simulink model "balanceActual"  (R2012b)
settings: Solver=ode3  StartTime=0.0  StopTime=inf  FixedStep=0.001  RelTol=1e-3
undefined symbols (not defined in the file or in its folder): HIL, qc_get_step_size
libraries: quarc_library x7
settings Model: SimulationMode=external  ExtModeTrigDuration=15000  Creator=runkunwang  LastModifiedBy=runkunwang
settings SolverCC: PositivePriorityOrder=on
settings RTWCC: SystemTargetFile=quarc_win64.tlc  TemplateMakefile=quarc_default_tmf  Description=QUARC Win64 Target  ProcessScript=quarc_win64_make_rtw_hook
settings STFCustomTargetCC: TargetPreCompLibLocation=C:\PROGRA~3\QUARC\lib\2012b\win64\release  CodeReplacementLibrary=ANSI_C  GeneratePreprocessorConditionals=Disable all  CombineOutputUpdateFcns=on  GRTInterface=off  SystemTargetFile=quarc_win64.tlc
settings GRTTargetCC: TargetPreCompLibLocation=C:\PROGRA~3\QUARC\lib\2012b\win64\release  ParMdlRefBuildCompliant=off  CompOptLevelCompliant=off  ConcurrentExecutionCompliant=off  MatFileLogging=off  ExtMode=on  ExtModeMexFile=quarc_comm

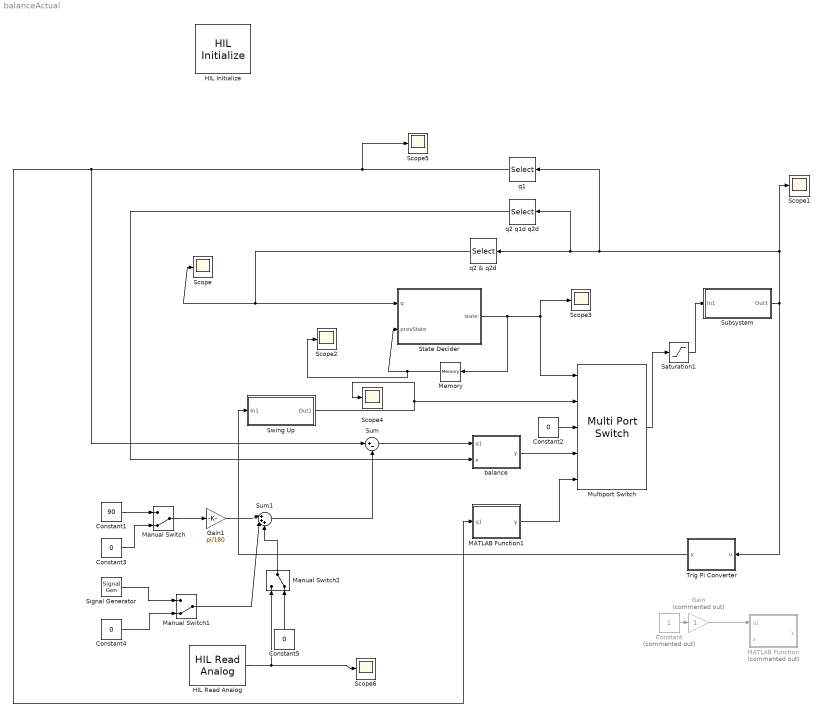
== system balanceActual ==
  Constant : Constant  Commented=on
  Constant1 : Constant  Value=90
  Constant{2..5} (4 alike) : Constant  Value=0
  Gain : Gain  Commented=on
  Gain1 : Gain  Gain=pi/180
  HIL Initialize : quarc_library/Data Acquisition/Generic/Configuration/HIL Initialize  Priority=-99  object_name=HIL-1  board_type=q2_usb  board_number=0  board_options=d0=digital;d1=digital;led=auto;update_rate=normal;decimation=1  exclusive=off  active=off  hardware_clocks=[0]  clock_modes=[]  initial_clock_frequencies=[]  set_clock_params_at_start=off  set_clock_params_at_switch_in=off  set_clock_frequencies_at_start=off  set_clock_frequencies_at_switch_in=off  analog_input_channels=[0:1]  analog_input_maximums=10  analog_input_minimums=-10  set_analog_input_params_at_start=on  set_analog_input_params_at_switch_in=off  analog_output_channels=[0:1]  analog_output_maximums=10  analog_output_minimums=-10  initial_analog_outputs=[0]  final_analog_outputs=[0]  watchdog_analog_outputs=0  set_analog_output_params_at_start=on  set_analog_output_params_at_switch_in=off  set_analog_outputs_at_start=on  set_analog_outputs_at_switch_in=off  set_analog_outputs_at_terminate=on  set_analog_outputs_at_switch_out=off  set_analog_outputs_on_watchdog=off  digital_input_channels=[]  digital_output_channels=[]  digital_output_configuration=[]  initial_digital_outputs=[1]  final_digital_outputs=[1]  watchdog_digital_outputs=[1]  set_digital_output_params_at_start=off  set_digital_output_params_at_switch_in=off  set_digital_outputs_at_start=on  set_digital_outputs_at_switch_in=off  set_digital_outputs_at_terminate=on  set_digital_outputs_at_switch_out=off  set_digital_outputs_on_watchdog=off  encoder_channels=[0:1]  quadrature=[4]  encoder_filter_frequency=[]  initial_encoder_counts=[0]  set_encoder_params_at_start=on  set_encoder_params_at_switch_in=off  set_encoder_counts_at_start=on  set_encoder_counts_at_switch_in=off  pwm_channels=[]  pwm_modes=[0]  pwm_frequency=1/0.020  pwm_configuration=[]  pwm_alignment=[]  pwm_polarity=[]  pwm_leading_deadband=[]  pwm_trailing_deadband=[]  initial_pwm_outputs=[0]  final_pwm_outputs=[0]  watchdog_pwm_outputs=[0]  set_pwm_params_at_start=on  set_pwm_params_at_switch_in=off  set_pwm_outputs_at_start=on  set_pwm_outputs_at_switch_in=off  set_pwm_outputs_at_terminate=on  set_pwm_outputs_at_switch_out=off  set_pwm_outputs_on_watchdog=off  other_output_channels=[]  initial_other_outputs=[]  final_other_outputs=[]  watchdog_other_outputs=[]  set_other_outputs_at_start=off  set_other_outputs_at_switch_in=off  set_other_outputs_at_terminate=off  set_other_outputs_at_switch_out=off  set_other_outputs_on_watchdog=off
  HIL Read Analog : quarc_library/Data Acquisition/Generic/Immediate I//O/HIL Read Analog  object_name=HIL-1  channels=0  sample_time=qc_get_step_size  active=on  vector_output=off
  MATLAB Function : MATLAB Function  Commented=on  TreatAsAtomicUnit=on
  MATLAB Function1 : MATLAB Function  TreatAsAtomicUnit=on
  Manual Switch : ManualSwitch  CurrentSetting=0
  Manual Switch1 : ManualSwitch  CurrentSetting=0
  Manual Switch2 : ManualSwitch  CurrentSetting=0
  Memory : Memory  X0=1
  Multiport Switch : MultiPortSwitch  Inputs=4
  Saturation1 : Saturate  UpperLimit=10  LowerLimit=-10
  Scope{,1..6} (7 alike) : Scope
      Scope settings: YMin=-0.5  YMax=9.5
      Scope1 settings: YMin=-0.6  YMax=0.7
      Scope2 settings: SaveName=ScopeData2  MaxDataPoints=10000
      Scope3 settings: SaveName=ScopeData3  MaxDataPoints=10000
      Scope4 settings: SaveName=ScopeData4  MaxDataPoints=10000
      Scope5 settings: YMin=-0.5  YMax=9.5  SaveName=ScopeData5
      Scope6 settings: SaveName=ScopeData6
  Signal Generator : SignalGenerator  Amplitude=50  Frequency=0.1
  State Decider : MATLAB Function  TreatAsAtomicUnit=on
  Subsystem : Subsystem
  Sum : Sum  Inputs=|+-
  Sum1 : Sum  Inputs=|+++
  Swing Up : Subsystem
  Trig Pi Converter : MATLAB Function  TreatAsAtomicUnit=on
  balance : MATLAB Function  TreatAsAtomicUnit=on
  q1 : Selector  InputPortWidth=4  IndexOptions=Index vector (dialog)  Indices=[1]  OutputSizes=1
  q2 & q2d : Selector  InputPortWidth=4  IndexOptions=Index vector (dialog)  Indices=[1 3 4]  OutputSizes=1
  q2 q1d q2d : Selector  InputPortWidth=4  IndexOptions=Index vector (dialog)  Indices=[2 3 4]  OutputSizes=1
  wires:
  State Decider/1(state) -> Memory/1, Multiport Switch/1, Scope3/1
  Constant2/1 -> Multiport Switch/3
  q2 & q2d/1 -> Scope/1, State Decider/1(q)
  Multiport Switch/1 -> Saturation1/1
  Saturation1/1 -> Subsystem/1(In1)
  Memory/1 -> Scope2/1, State Decider/2(prevState)
  Swing Up/1(Out1) -> Scope4/1, Multiport Switch/2
  Subsystem/1(Out1) -> Trig Pi Converter/1(u), Scope1/1, q1/1, q2 q1d q2d/1, q2 & q2d/1
  Trig Pi Converter/1(y) -> Swing Up/1(In1)
  balance/1(y) -> Multiport Switch/4
  Constant/1 -> Gain/1
  Gain/1 -> MATLAB Function/1(q1)
  q2 q1d q2d/1 -> balance/2(x)
  q1/1 -> MATLAB Function1/1(q1), Sum/1, Scope5/1
  Sum/1 -> balance/1(q1)
  Constant1/1 -> Manual Switch/1
  Constant3/1 -> Manual Switch/2
  Signal Generator/1 -> Manual Switch1/1
  Constant4/1 -> Manual Switch1/2
  Manual Switch1/1 -> Sum1/2
  MATLAB Function1/1(y) -> Multiport Switch/5
  Manual Switch/1 -> Gain1/1
  Gain1/1 -> Sum1/1
  Sum1/1 -> Sum/2
  HIL Read Analog/1 -> Manual Switch2/1, Scope6/1
  Manual Switch2/1 -> Sum1/3
  Constant5/1 -> Manual Switch2/2

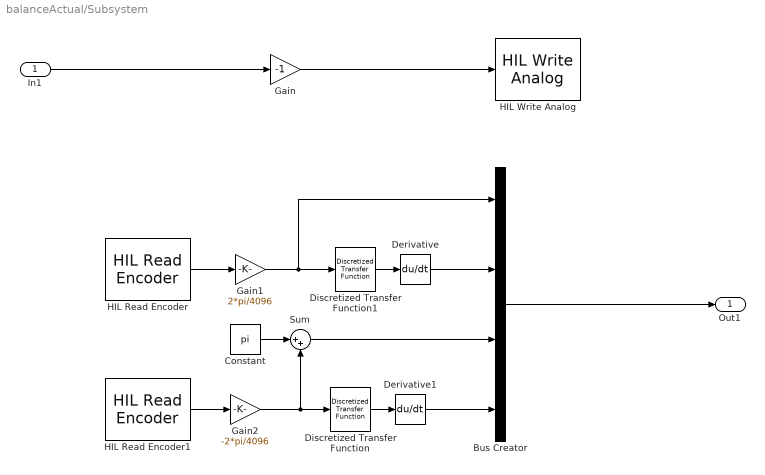
== system balanceActual/Subsystem ==
  In1 : Inport
  Bus Creator : BusCreator
  Constant : Constant  Value=pi
  Derivative : Derivative
  Derivative1 : Derivative
  Discretized Transfer Function : quarc_library/Discrete/Discretized Transfer Function  num=100  den=[1 100]  method=tustin  Ts=qc_get_step_size
  Discretized Transfer Function1 : quarc_library/Discrete/Discretized Transfer Function  num=100  den=[1 100]  method=tustin  Ts=qc_get_step_size
  Gain : Gain  Gain=-1
  Gain1 : Gain  Gain=2*pi/4096  ParamMin=[-512]  ParamMax=[512]
  Gain2 : Gain  Gain=-2*pi/4096  ParamMin=[-512]  ParamMax=[512]
  HIL Read Encoder : quarc_library/Data Acquisition/Generic/Immediate I//O/HIL Read Encoder  object_name=HIL-1  channels=0  sample_time=qc_get_step_size  active=on  vector_output=off  data_type_mode=Inherit via back propagation  data_type=double
  HIL Read Encoder1 : quarc_library/Data Acquisition/Generic/Immediate I//O/HIL Read Encoder  object_name=HIL-1  channels=1  sample_time=qc_get_step_size  active=on  vector_output=off  data_type_mode=Inherit via back propagation  data_type=double
  HIL Write Analog : quarc_library/Data Acquisition/Generic/Immediate I//O/HIL Write Analog  object_name=HIL-1  channels=0  sample_time=-1  active=off  vector_input=off
  Sum : Sum  Inputs=|++
  Out1 : Outport
  wires:
  HIL Read Encoder/1 -> Gain1/1
  HIL Read Encoder1/1 -> Gain2/1
  Gain1/1 -> Bus Creator/1, Discretized Transfer Function1/1
  Gain2/1 -> Discretized Transfer Function/1, Sum/2
  Discretized Transfer Function1/1 -> Derivative/1
  Discretized Transfer Function/1 -> Derivative1/1
  Constant/1 -> Sum/1
  In1/1 -> Gain/1
  Gain/1 -> HIL Write Analog/1
  Bus Creator/1 -> Out1/1
  Derivative/1 -> Bus Creator/2
  Sum/1 -> Bus Creator/3
  Derivative1/1 -> Bus Creator/4

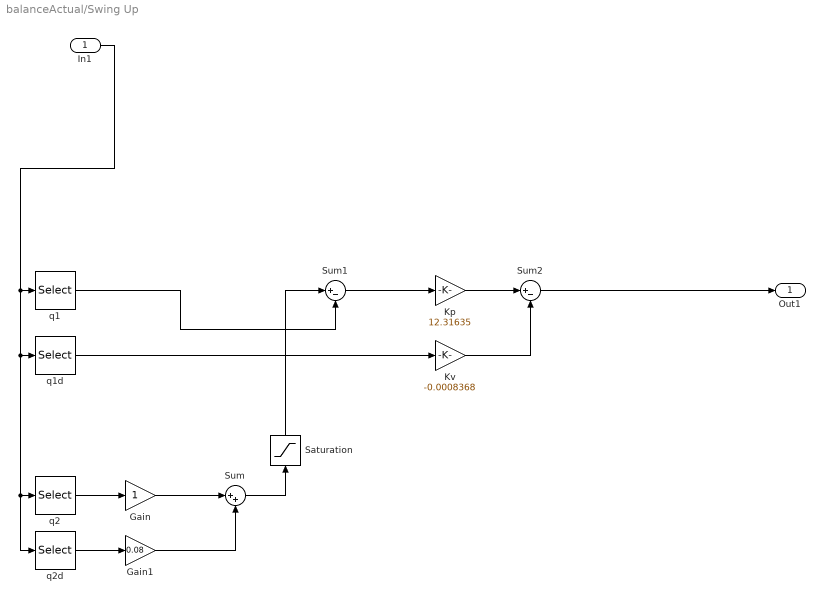
== system balanceActual/Swing Up ==
  In1 : Inport
  Gain : Gain
  Gain1 : Gain  Gain=0.08
  Kp : Gain  Gain=12.31635
  Kv : Gain  Gain=-0.0008368
  Saturation : Saturate
  Sum : Sum  Inputs=|++
  Sum1 : Sum  Inputs=|+-
  Sum2 : Sum  Inputs=|+-
  q1 : Selector  InputPortWidth=4  IndexOptions=Index vector (dialog)  Indices=[1]  OutputSizes=1
  q1d : Selector  InputPortWidth=4  IndexOptions=Index vector (dialog)  Indices=[2]  OutputSizes=1
  q2 : Selector  InputPortWidth=4  IndexOptions=Index vector (dialog)  Indices=[3]  OutputSizes=1
  q2d : Selector  InputPortWidth=4  IndexOptions=Index vector (dialog)  Indices=[4]  OutputSizes=1
  Out1 : Outport
  wires:
  In1/1 -> q2d/1, q2/1, q1d/1, q1/1
  q1d/1 -> Kv/1
  q2/1 -> Gain/1
  q2d/1 -> Gain1/1
  Gain/1 -> Sum/1
  Gain1/1 -> Sum/2
  Sum1/1 -> Kp/1
  Kv/1 -> Sum2/2
  Kp/1 -> Sum2/1
  Sum2/1 -> Out1/1
  Sum/1 -> Saturation/1
  q1/1 -> Sum1/2
  Saturation/1 -> Sum1/1

== matlab function balanceActual/Trig Pi Converter ==
  data: u input; y output
function y = fcn(u)
q1 = u(1);
q1d = u(2);
q2d = u(4);
q2 = u(3);
q2 = q2 - pi;
y = [q1 q1d atan2(sin(q2),cos(q2)) q2d];

== matlab function balanceActual/State Decider ==
  data: q input; state output; prevState input
function state = fcn(q, prevState)
q1 = q(1);
q2 = q(2);
q2d = q(3);
q2 = q2 - pi;

%q1 mod
if q1 < 0
    q1 = -q1;
end
if q1 > 2*pi
    q1 = mod(q1, 2*pi);
end

%q2 mod
if q2 < 0
    q2 = -q2;
end
if q2 > 2*pi
    q2 = mod(q2, 2*pi);
end

%controller starts
%Zone 1 to Zone 3
if prevState == 1 && (q2 > (8*pi)/9 && q2 < (10*pi)/9)
    %Zone 3
    state = 3;
%Zone 3 to Zone 2
elseif prevState == 3 && (q2 < (8*pi)/9 || q2 > (10*pi)/9)
    %Zone 2
    state = 2; 
%Fourth State to Zone 1
elseif prevState == 4 && (q2 < (pi/18) && q2 < (35*pi/18)) && (abs(q2d) < 1) && (q1 < pi/18 || q1 > 35*pi/18)
    %Zone 1
    state = 1; 

%fourth state
elseif prevState == 2 && (q2 < (pi/18) && q2 < (35*pi/18)) && (abs(q2d) < 1) && q1 ~= 0
    %State 4
    state = 4;
%Zone 2 to Zone 1
    
else state = prevState;
end

end

== matlab function balanceActual/MATLAB Function ==
  data: q1 input; y output; x input
function y = fcn(q1, x)

%theta values
t1 = 0.0790;
t2 = 0.0277;
t3 = 0.0278;
t4 = 0.1347;
t5 = 0.5397;
t6 = 0.0057;

%actual position
q1a = x(1);
q2a = x(3);
q1da = x(2);
q2da = x(4);
q2n = atan2(sin(q2a),cos(q2a));

%desired positions
q2 = 0;
q1d = 0;
q2d = 0;
%A matrx
A = zeros(4);
A(1,2) = 1;
A(3,4) = 1;
A(2,2) = - (t2*(t5 + 2*q2d*t2*cos(q2)*sin(q2)))/(t1*t2 - t3^2*cos(q2)^2 + t2^2*sin(q2)^2) - (2*q1d*t2*t3*cos(q2)^2*sin(q2))/(t1*t2 - t3^2*cos(q2)^2 + t2^2*sin(q2)^2);
A(2,3) = (t2*(q2d^2*t3*cos(q2) - 2*q1d*q2d*t2*cos(q2)^2 + 2*q1d*q2d*t2*sin(q2)^2))/(t1*t2 - t3^2*cos(q2)^2 + t2^2*sin(q2)^2) - (t3*cos(q2)*((981*t4*cos(q2))/100 + q1d^2*t2*cos(q2)^2 - q1d^2*t2*sin(q2)^2))/(t1*t2 - t3^2*cos(q2)^2 + t2^2*sin(q2)^2) + (t3*sin(q2)*(t2*cos(q2)*sin(q2)*q1d^2 - q2d*t6 + (981*t4*sin(q2))/100))/(t1*t2 - t3^2*cos(q2)^2 + t2^2*sin(q2)^2) - (t2*(2*cos(q2)*sin(q2)*t2^2 + 2*cos(q2)*sin(q2)*t3^2)*(t3*sin(q2)*q2d^2 - 2*q1d*t2*cos(q2)*sin(q2)*q2d + v - q1d*t5))/(t2^2*sin(q2)^2 + t1*t2 - t3^2*cos(q2)^2)^2 + (t3*cos(q2)*(2*cos(q2)*sin(q2)*t2^2 + 2*cos(q2)*sin(q2)*t3^2)*(t2*cos(q2)*sin(q2)*q1d^2 - q2d*t6 + (981*t4*sin(q2))/100))/(t2^2*sin(q2)^2 + t1*t2 - t3^2*cos(q2)^2)^2;
A(2,4) = (cos(q2)*(- 2*q1d*sin(q2)*t2^2 + t3*t6) + 2*q2d*t2*t3*sin(q2))/(t1*t2 - t3^2*cos(q2)^2 + t2^2*sin(q2)^2);
A(4,2) = (cos(q2)*(2*q1d*t2^2*sin(q2)^3 + 2*q1d*t1*t2*sin(q2)) + t3*cos(q2)*(t5 + 2*q2d*t2*cos(q2)*sin(q2)))/(t1*t2 - t3^2*cos(q2)^2 + t2^2*sin(q2)^2);
A(4,3) = ((t2*sin(q2)^2 + t1)*((981*t4*cos(q2))/100 + q1d^2*t2*cos(q2)^2 - q1d^2*t2*sin(q2)^2))/(t1*t2 - t3^2*cos(q2)^2 + t2^2*sin(q2)^2) - ((2*cos(q2)*sin(q2)*t2^2 + 2*cos(q2)*sin(q2)*t3^2)*(t2*sin(q2)^2 + t1)*(t2*cos(q2)*sin(q2)*q1d^2 - q2d*t6 + (981*t4*sin(q2))/100))/(t2^2*sin(q2)^2 + t1*t2 - t3^2*cos(q2)^2)^2 - (t3*cos(q2)*(q2d^2*t3*cos(q2) - 2*q1d*q2d*t2*cos(q2)^2 + 2*q1d*q2d*t2*sin(q2)^2))/(t1*t2 - t3^2*cos(q2)^2 + t2^2*sin(q2)^2) + (t3*sin(q2)*(t3*sin(q2)*q2d^2 - 2*q1d*t2*cos(q2)*sin(q2)*q2d + v - q1d*t5))/(t1*t2 - t3^2*cos(q2)^2 + t2^2*sin(q2)^2) + (2*t2*cos(q2)*sin(q2)*(t2*cos(q2)*sin(q2)*q1d^2 - q2d*t6 + (981*t4*sin(q2))/100))/(t1*t2 - t3^2*cos(q2)^2 + t2^2*sin(q2)^2) + (t3*cos(q2)*(2*cos(q2)*sin(q2)*t2^2 + 2*cos(q2)*sin(q2)*t3^2)*(t3*sin(q2)*q2d^2 - 2*q1d*t2*cos(q2)*sin(q2)*q2d + v - q1d*t5))/(t2^2*sin(q2)^2 + t1*t2 - t3^2*cos(q2)^2)^2;
A(4,4) = -(t1*t6 + t2*(t6*sin(q2)^2 - 2*q1d*t3*cos(q2)^2*sin(q2)) + 2*q2d*t3^2*cos(q2)*sin(q2))/(t1*t2 - t3^2*cos(q2)^2 + t2^2*sin(q2)^2);

%B matrix 
B =  [0; t2/(- t3^2 + t1*t2); 0; -t3/(- t3^2 + t1*t2)];

%K 
K = place(A,B, [-5 -5.1 -5.2 -5.3]);
u = -K*[q1a; q1da; q2n; q2da];

y = u;

== matlab function balanceActual/balance ==
  data: q1 input; x input; y output
function y = fcn(q1, x)
q2 = x(2);
q1d = x(1);
q2d = x(3);
q2n = atan2(sin(q2),cos(q2));
K = [-0.7528   -1.1279  -12.7270   -1.6188];
u = -K*[q1; q1d; q2n; q2d];
y = u;

== matlab function balanceActual/MATLAB Function1 ==
  data: q1 input; y output
function y = fcn(q1)
%#codegen
%k = -0.7528
k = -1;
y = q1*k;
